simulink model "MPCRLpredict"  (R2023a)
settings: Solver=ode1  StartTime=0.0  StopTime=inf  FixedStep=0.005  RelTol=1e-3  EnableMultiTasking=on
values from neighbouring files (symbols this model uses):
  B = -100    [RLmpcTrainPredict.m]
  bp = 5e-5*2    (= 0.0001)    [Copy_of_qube2_rotpen_param.m]    (also in MPCmodelinitial.m = 5e-05)
  br = 1e-3*2    (= 0.002)    [Copy_of_qube2_rotpen_param.m]    (also in MPCmodelinitial.m = 0.001)
  g = 9.81    [Copy_of_qube2_rotpen_param.m]    (also in MPCmodelinitial.m)
  Jp = mp*Lp^2/3    (= 0.0001464408)    [Copy_of_qube2_rotpen_param.m]    (also in MPCmodelinitial.m = 0.000133128)
  Jr = mr*r^2/3    (= 0.000251670833333)    [Copy_of_qube2_rotpen_param.m]    (also in MPCmodelinitial.m = 0.000228791666667)
  km = kt    (= 0.042)    [Copy_of_qube2_rotpen_param.m]    (also in MPCmodelinitial.m)
  kt = 0.042    [Copy_of_qube2_rotpen_param.m]    (also in MPCmodelinitial.m)
  l = Lp/2    (= 0.0645)    [Copy_of_qube2_rotpen_param.m]    (also in MPCmodelinitial.m)
  mp = 0.024*1.1    (= 0.0264)    [Copy_of_qube2_rotpen_param.m]    (also in MPCmodelinitial.m = 0.024)
  q11 = 5    [RLmpcTrainPredict.m]
  q22 = 5    [RLmpcTrainPredict.m]
  q33 = 0    [RLmpcTrainPredict.m]
  q44 = 0    [RLmpcTrainPredict.m]
  r = 0.085    [Copy_of_qube2_rotpen_param.m]    (also in MPCmodelinitial.m)
  Rm = 9.7    [Copy_of_qube2_rotpen_param.m]    (also in MPCmodelinitial.m = 8.4)
  theta_max = 2    [RLmpcTrainPredict.m]
  UR = 0.1    [RLmpcTrainPredict.m]
  UVR = 0    [RLmpcTrainPredict.m]
undefined symbols (not defined in the file or in its folder): ic_alpha0
libraries: simulink x5, mpclib x1, rllib x1, sdolib x1
settings Model: ExtModeTrigDuration=10000  Creator=XIJ62  LastModifiedBy=XIJ62
settings SolverCC: AlgebraicLoopSolver=TrustRegion  PositivePriorityOrder=on
settings DataIOCC: ReturnWorkspaceOutputs=off
settings DebuggingCC: UnconnectedInputMsg=warning  UnconnectedOutputMsg=warning  UnconnectedLineMsg=warning  ArithmeticOperatorsInVariantConditions=warning
settings ModelReferenceCC: EnableRefExpFcnMdlSchedulingChecks=on
settings SFSimCC: SimUseLocalCustomCode=off  CustomCodeUndefinedFunction=UseInterfaceOnly
settings RTWCC: Description=QUARC Win64 Target Using Toolchain  SystemTargetFile=quarc_win64.tlc  TemplateMakefile=quarc_default_tmf  RTWUseLocalCustomCode=off  Toolchain=QUARC win64 | nmake (64-bit Windows)  BuildConfiguration=Faster Runs  DLArmComputeVersion=19.05
settings CodeAppCC: StateflowObjectComments=on
settings STFCustomTargetCC: SystemTargetFile=quarc_win64.tlc
settings GRTTargetCC: ParMdlRefBuildCompliant=off  CompOptLevelCompliant=off  CombineOutputUpdateFcns=off  MatFileLogging=off  CPPClassGenCompliant=off  GRTInterface=on  ExtMode=on  ExtModeMexFile=quarc_comm
settings ConfigComp: CovMetricSettings=dswe

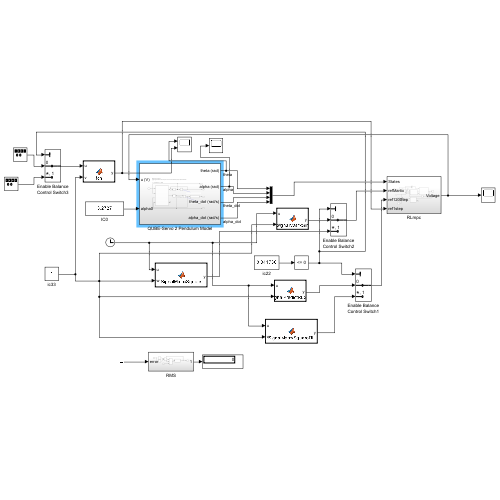
[thumbnail: Simulink's stored preview of the top-level diagram]
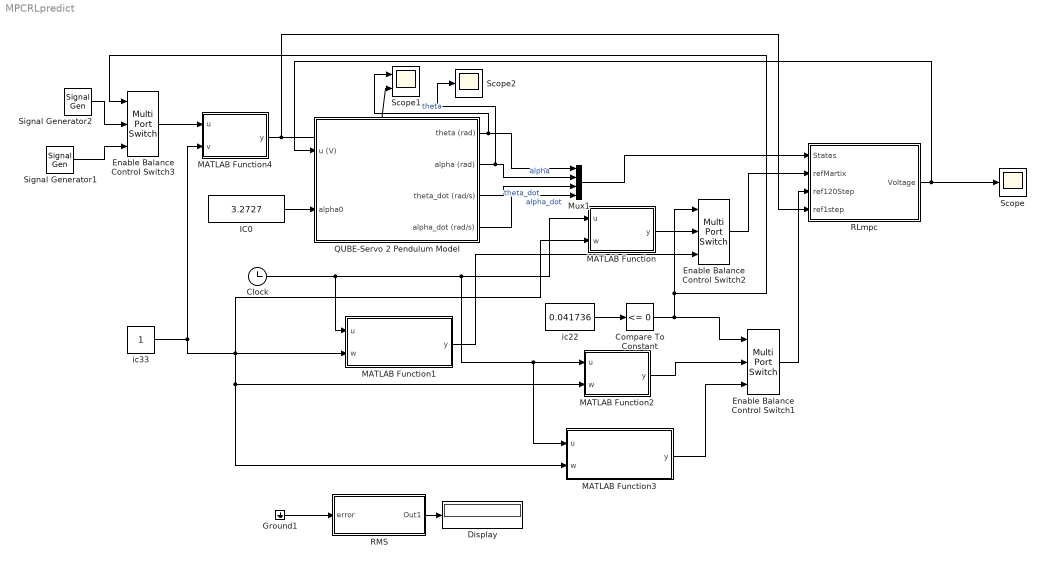
== system MPCRLpredict ==
  Clock : Clock
  Compare To Constant : simulink/Logic and Bit Operations/Compare To Constant  relop=<=  const=0  OutDataTypeStr=boolean
  Display : Display
  Enable Balance Control Switch1 : MultiPortSwitch  DataPortOrder=Zero-based contiguous  Inputs=2  zeroidx=on  SaturateOnIntegerOverflow=off  InputSameDT=off
  Enable Balance Control Switch2 : MultiPortSwitch  DataPortOrder=Zero-based contiguous  Inputs=2  zeroidx=on  SaturateOnIntegerOverflow=off  InputSameDT=off
  Enable Balance Control Switch3 : MultiPortSwitch  DataPortOrder=Zero-based contiguous  Inputs=2  zeroidx=on  SaturateOnIntegerOverflow=off  InputSameDT=off
  Ground1 : Ground
  IC0 : Constant  Value=3.2727
  MATLAB Function : MATLAB Function  TreatAsAtomicUnit=on
  MATLAB Function1 : MATLAB Function  TreatAsAtomicUnit=on
  MATLAB Function2 : MATLAB Function  TreatAsAtomicUnit=on
  MATLAB Function3 : MATLAB Function  TreatAsAtomicUnit=on
  MATLAB Function4 : MATLAB Function  TreatAsAtomicUnit=on
  Mux1 : Mux
  QUBE-Servo 2 Pendulum Model : Subsystem
  RLmpc : Subsystem
  RMS : Subsystem
  Scope : Scope
  Scope1 : Scope  NumInputPorts=2
  Scope2 : Scope
  Signal Generator1 : SignalGenerator  WaveForm=square  Amplitude=0.5  Units=rad/sec
  Signal Generator2 : SignalGenerator  Units=rad/sec
  ic22 : Constant  Value=0.041736
  ic33 : Constant
  wires:
  RLmpc/1(Voltage) -> Scope/1, QUBE-Servo 2 Pendulum Model/1(u (V))
  Signal Generator1/1 -> Enable Balance Control Switch3/3
  Clock/1 -> MATLAB Function/1(u), MATLAB Function3/1(u), MATLAB Function2/1(u), MATLAB Function1/1(u)
  MATLAB Function1/1(y) -> Enable Balance Control Switch2/3
  QUBE-Servo 2 Pendulum Model/1(theta (rad)) -> Scope1/1, Mux1/1  "theta"
  QUBE-Servo 2 Pendulum Model/2(alpha (rad)) -> Scope2/1, Mux1/2  "alpha"
  QUBE-Servo 2 Pendulum Model/3(theta_dot (rad/s)) -> Mux1/3  "theta_dot"
  QUBE-Servo 2 Pendulum Model/4(alpha_dot (rad/s)) -> Mux1/4  "alpha_dot"
  Mux1/1 -> RLmpc/1(States)
  IC0/1 -> QUBE-Servo 2 Pendulum Model/2(alpha0)
  RMS/1(Out1) -> Display/1
  Ground1/1 -> RMS/1(error)
  MATLAB Function2/1(y) -> Enable Balance Control Switch1/2
  Enable Balance Control Switch1/1 -> RLmpc/3(ref120Step)
  MATLAB Function3/1(y) -> Enable Balance Control Switch1/3
  Compare To Constant/1 -> Enable Balance Control Switch3/1, Enable Balance Control Switch2/1, Enable Balance Control Switch1/1
  ic22/1 -> Compare To Constant/1
  MATLAB Function/1(y) -> Enable Balance Control Switch2/2
  Enable Balance Control Switch2/1 -> RLmpc/2(refMartix)
  Signal Generator2/1 -> Enable Balance Control Switch3/2
  ic33/1 -> MATLAB Function4/2(v), MATLAB Function3/2(w), MATLAB Function2/2(w), MATLAB Function1/2(w), MATLAB Function/2(w)
  Enable Balance Control Switch3/1 -> MATLAB Function4/1(u)
  MATLAB Function4/1(y) -> Scope1/2, RLmpc/4(ref1step)

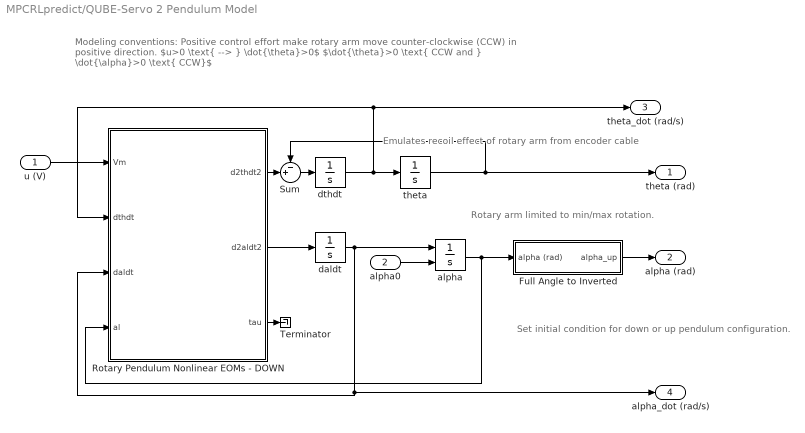
== system MPCRLpredict/QUBE-Servo 2 Pendulum Model ==
  note: Rotary arm limited to min/max rotation.
  note: Modeling conventions:
      | Positive control effort make rotary arm move counter-clockwise (CCW) in positive direction.
      | $u>0 \text{ --> } \dot{\theta}>0$
      | $\dot{\theta}>0 \text{ CCW and } \dot{\alpha}>0 \text{ CCW}$
  note: Set initial condition for down or up pendulum configuration.
  note: Emulates recoil effect of rotary arm from encoder cable
  u (V) : Inport
  alpha0 : Inport  Port=2
  Full Angle to Inverted : Subsystem
  Rotary Pendulum Nonlinear EOMs - DOWN : MATLAB Function  TreatAsAtomicUnit=on
  Sum : Sum  Inputs=-+|
  Terminator : Terminator
  alpha : Integrator  InitialConditionSource=external  InitialCondition=ic_alpha0
  daldt : Integrator
  dthdt : Integrator
  theta : Integrator  LimitOutput=on  UpperSaturationLimit=theta_max  LowerSaturationLimit=-theta_max
  theta (rad) : Outport  VectorParamsAs1DForOutWhenUnconnected=off
  alpha (rad) : Outport  Port=2  VectorParamsAs1DForOutWhenUnconnected=off
  theta_dot (rad/s) : Outport  Port=3  VectorParamsAs1DForOutWhenUnconnected=off
  alpha_dot (rad/s) : Outport  Port=4  VectorParamsAs1DForOutWhenUnconnected=off
  wires:
  daldt/1 -> Rotary Pendulum Nonlinear EOMs - DOWN/3(daldt), alpha_dot (rad/s)/1, alpha/1
  alpha/1 -> Full Angle to Inverted/1(alpha (rad)), Rotary Pendulum Nonlinear EOMs - DOWN/4(al)
  Rotary Pendulum Nonlinear EOMs - DOWN/2(d2aldt2) -> daldt/1
  dthdt/1 -> theta_dot (rad/s)/1, Rotary Pendulum Nonlinear EOMs - DOWN/2(dthdt), theta/1
  u (V)/1 -> Rotary Pendulum Nonlinear EOMs - DOWN/1(Vm)
  Rotary Pendulum Nonlinear EOMs - DOWN/3(tau) -> Terminator/1
  Full Angle to Inverted/1(alpha_up) -> alpha (rad)/1
  alpha0/1 -> alpha/2
  theta/1 -> theta (rad)/1, Sum/1
  Rotary Pendulum Nonlinear EOMs - DOWN/1(d2thdt2) -> Sum/2
  Sum/1 -> dthdt/1

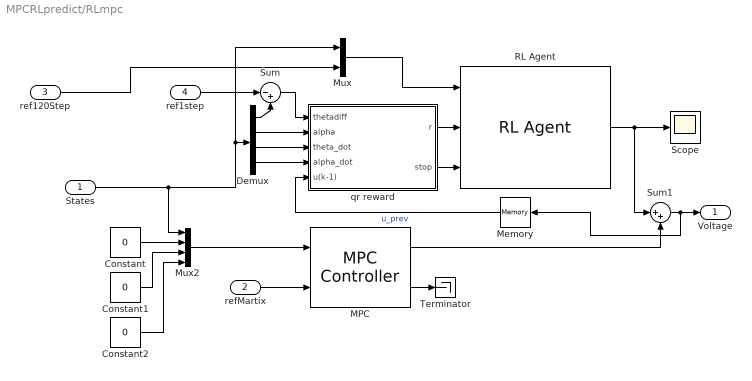
== system MPCRLpredict/RLmpc ==
  States : Inport
  refMartix : Inport  Port=2
  ref120Step : Inport  Port=3
  ref1step : Inport  Port=4
  Constant : Constant  Value=0
  Constant1 : Constant  Value=0
  Constant2 : Constant  Value=0
  Demux : Demux
  MPC : mpclib/MPC Controller  SCDEnableBlockLinearizationSpecification=on  mpcobj=mpc1  is_multiple=0  enable_value=0  return_u0=off  updateMPCinCallerWorkspace=on  md_inport=off  mv_inport=off  uref_inport=off  return_cost=off  return_mvseq=off  return_qpstatus=off  return_xseq=off  return_state=on  return_ovseq=off  state_inport=on  umin_inport=off  umax_inport=off  ymin_inport=off  ymax_inport=off  cc_inport=off  ywt_inport=off  uwt_inport=off  duwt_inport=off  rhoeps_inport=off  pm_inport=off  MaximumP=10  HorizonChoice=FixedHorizon  n_ts=0.005  n_p=120  n_mv=1  n_md=0  n_ud=0  n_mo=4  n_uo=0  BlockDataType=double  SampleTimeInherited=off  switch_inport=off
  Memory : Memory
  Mux : Mux  Inputs=2
  Mux2 : Mux
  RL Agent : rllib/RL Agent  Agent=agent  ExternalActionAsInput=off  ProvideLastAction=off  ProvideCumRwd=off  TreatAsDirectFeedthrough=on  UseStrictObservationDataTypes=off
  Scope : Scope
  Sum : Sum  Inputs=|-+
  Sum1 : Sum  Inputs=|++
  Terminator : Terminator
  qr reward : Subsystem
  Voltage : Outport
  wires:
  States/1 -> Mux2/1, Mux/1, Demux/1
  refMartix/1 -> MPC/2
  qr reward/2(stop) -> RL Agent/3
  qr reward/1(r) -> RL Agent/2
  Demux/2 -> qr reward/2(alpha)
  Demux/3 -> qr reward/3(theta_dot)
  Demux/4 -> qr reward/4(alpha_dot)
  Demux/1 -> Sum/2
  Sum/1 -> qr reward/1(thetadiff)
  Mux/1 -> RL Agent/1
  RL Agent/1 -> Sum1/1, Scope/1
  Memory/1 -> qr reward/5(u(k-1))  "u_prev"
  MPC/2 -> Terminator/1
  MPC/1 -> Sum1/2
  Sum1/1 -> Memory/1, Voltage/1
  Constant1/1 -> Mux2/3
  Constant2/1 -> Mux2/4
  Constant/1 -> Mux2/2
  Mux2/1 -> MPC/1
  ref120Step/1 -> Mux/2
  ref1step/1 -> Sum/1

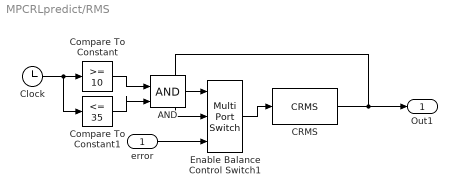
== system MPCRLpredict/RMS ==
  error : Inport
  AND : Logic  IconShape=distinctive  AllPortsSameDT=off  OutDataTypeStr=boolean
  CRMS : sdolib/RMS Blocks/CRMS
  Clock : Clock
  Compare To Constant : simulink/Logic and Bit Operations/Compare To Constant  relop=>=  const=10  OutDataTypeStr=boolean
  Compare To Constant1 : simulink/Logic and Bit Operations/Compare To Constant  relop=<=  const=35  OutDataTypeStr=boolean
  Enable Balance Control Switch1 : MultiPortSwitch  DataPortOrder=Zero-based contiguous  Inputs=2  zeroidx=on  SaturateOnIntegerOverflow=off  InputSameDT=off
  Out1 : Outport
  wires:
  Clock/1 -> Compare To Constant/1, Compare To Constant1/1
  Compare To Constant1/1 -> AND/2
  Compare To Constant/1 -> AND/1
  AND/1 -> Enable Balance Control Switch1/1
  Enable Balance Control Switch1/1 -> CRMS/1
  CRMS/1 -> Enable Balance Control Switch1/2, Out1/1
  error/1 -> Enable Balance Control Switch1/3

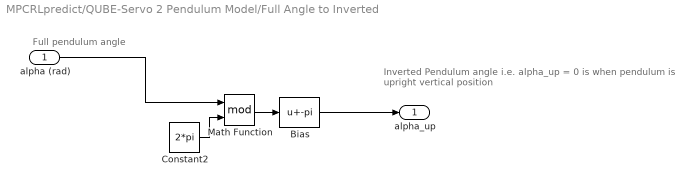
== system MPCRLpredict/QUBE-Servo 2 Pendulum Model/Full Angle to Inverted ==
  note: Inverted Pendulum angle
      | i.e. alpha_up = 0 is when pendulum is upright vertical position
  note: Full pendulum angle
  alpha (rad) : Inport
  Bias : Bias  Bias=-pi  SaturateOnIntegerOverflow=off
  Constant2 : Constant  Value=2*pi
  Math Function : Math  Operator=mod  SignedPower=on
  alpha_up : Outport  VectorParamsAs1DForOutWhenUnconnected=off
  wires:
  Constant2/1 -> Math Function/2
  Bias/1 -> alpha_up/1
  alpha (rad)/1 -> Math Function/1
  Math Function/1 -> Bias/1

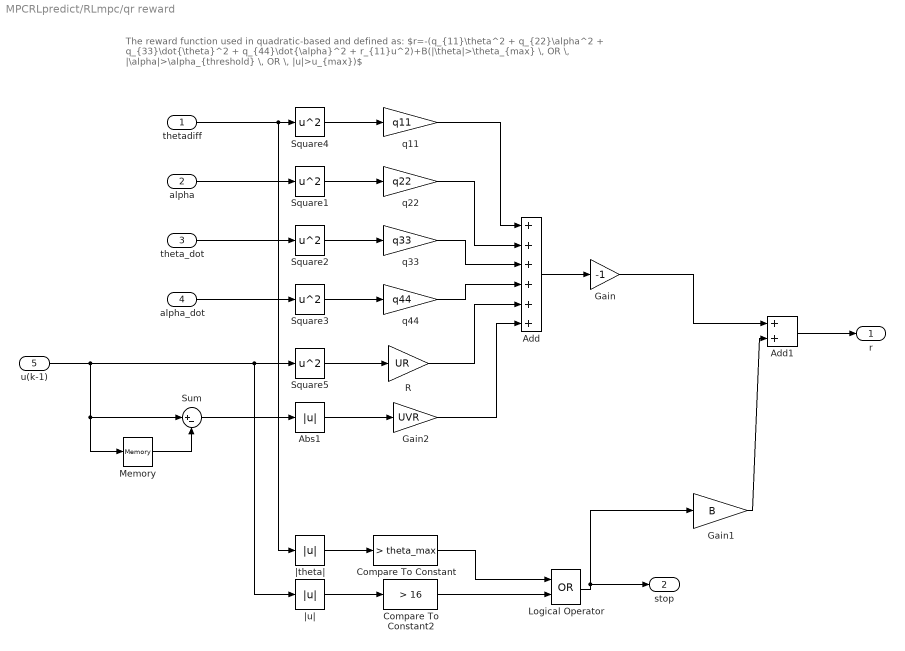
== system MPCRLpredict/RLmpc/qr reward ==
  note: The reward function used in quadratic-based and defined as:
      | $r=-(q_{11}\theta^2 + q_{22}\alpha^2 + q_{33}\dot{\theta}^2 + q_{44}\dot{\alpha}^2 + r_{11}u^2)+B(|\theta|>\theta_{max} \, OR \, |\alpha|>\alpha_{threshold} \, OR \, |u|>u_{max})$
  thetadiff : Inport
  alpha : Inport  Port=2
  theta_dot : Inport  Port=3
  alpha_dot : Inport  Port=4
  u(k-1) : Inport  Port=5
  Abs1 : Abs  SaturateOnIntegerOverflow=off
  Add : Sum  Inputs=++++++
  Add1 : Sum
  Compare To Constant : simulink/Logic and Bit Operations/Compare To Constant  relop=>  const=theta_max  OutDataTypeStr=boolean
  Compare To Constant2 : simulink/Logic and Bit Operations/Compare To Constant  relop=>  const=16  OutDataTypeStr=boolean
  Gain : Gain  Gain=-1
  Gain1 : Gain  Gain=B
  Gain2 : Gain  Gain=UVR
  Logical Operator : Logic  Operator=OR  AllPortsSameDT=off  OutDataTypeStr=boolean
  Memory : Memory
  R : Gain  Gain=UR
  Square{1..5} (5 alike) : Math  Operator=square
  Sum : Sum  Inputs=|+-
  q11 : Gain  Gain=q11
  q22 : Gain  Gain=q22
  q33 : Gain  Gain=q33
  q44 : Gain  Gain=q44
  |theta| : Abs  SaturateOnIntegerOverflow=off
  |u| : Abs  SaturateOnIntegerOverflow=off
  r : Outport  VectorParamsAs1DForOutWhenUnconnected=off
  stop : Outport  Port=2  VectorParamsAs1DForOutWhenUnconnected=off
  wires:
  |theta|/1 -> Compare To Constant/1
  thetadiff/1 -> Square4/1, |theta|/1
  Compare To Constant/1 -> Logical Operator/1
  alpha/1 -> Square1/1
  Logical Operator/1 -> Gain1/1, stop/1
  Square4/1 -> q11/1
  Square1/1 -> q22/1
  Square2/1 -> q33/1
  theta_dot/1 -> Square2/1
  alpha_dot/1 -> Square3/1
  Square3/1 -> q44/1
  u(k-1)/1 -> Square5/1, |u|/1, Sum/1, Memory/1
  Square5/1 -> R/1
  |u|/1 -> Compare To Constant2/1
  R/1 -> Add/5
  q11/1 -> Add/1
  q33/1 -> Add/3
  q22/1 -> Add/2
  q44/1 -> Add/4
  Add/1 -> Gain/1
  Compare To Constant2/1 -> Logical Operator/2
  Gain/1 -> Add1/1
  Gain1/1 -> Add1/2
  Add1/1 -> r/1
  Memory/1 -> Sum/2
  Sum/1 -> Abs1/1
  Abs1/1 -> Gain2/1
  Gain2/1 -> Add/6

== matlab function MPCRLpredict/MATLAB Function1 ==
  data: u input; y output; w input
function y = SignalMatrixSquare(u,w)
    Signal=zeros(120,4);
    for (k=1:120)
        t=floor((u+0.005*k-0.005)/pi);
        Signal(k,1)=mod(t,2)-0.5;
    end
    y = Signal*w;
end

== matlab function MPCRLpredict/MATLAB Function ==
  data: u input; y output; w input
function y = SignalMatrixSin(u,w)
    Np=120; %Prediction horizon
    Signal=zeros(120,4);
    t=u;
    for (k=1:120)
        Signal(k,1)=sin(t+0.005*k-0.005);
    end
    y = Signal*w;
end

== matlab function MPCRLpredict/MATLAB Function2 ==
  data: u input; y output; w input
function y = SignalPredictRLSin(u,w)
    Np=120; %Prediction horizon
    Signal=zeros(120,1);
    t=u;
    for (k=1:120)
        Signal(k)=sin(t+0.005*k-0.005);
    end
    y = Signal*w;
end

== matlab function MPCRLpredict/MATLAB Function3 ==
  data: u input; y output; w input
function y = SignalMatrixSquareRL(u,w)
    Signal=zeros(120,1);
    for (k=1:120)
        t=floor((u+0.005*k-0.005)/pi);
        Signal(k)=mod(t,2)-0.5;
    end
    y = Signal*w;
end

== matlab function MPCRLpredict/MATLAB Function4 ==
  data: u input; y output; v input
function y = fcn(u,v)
    
    
y=u*v;

== matlab function MPCRLpredict/QUBE-Servo 2 Pendulum Model/Rotary Pendulum Nonlinear EOMs - DOWN ==
  data: Vm input size=1; d2thdt2 output size=1; d2aldt2 output size=1; dthdt input size=1; daldt input size=1; Jp parameter; Jr parameter; l parameter; mp parameter; br parameter; bp parameter; r parameter; kt parameter; km parameter; Rm parameter; al input size=1; g parameter; tau output
function [d2thdt2,d2aldt2,tau] = pen_nonlin_eoms(Vm, dthdt, daldt, Jp, Jr, l, mp, br, bp, r, kt, km, Rm, al, g)

% Convert voltage to torque input
tau = (Vm - km*dthdt)/Rm;
tau=kt*tau;
% Denominator
Jt = Jr*Jp + Jp^2*sin(al)^2 - mp^2*r^2*l^2*cos(al)^2;
% Nonlinear equations of motion for generic rotary pendulum (i.e. furuta)
% Terms from EOM solving
term1 = tau - br*dthdt + 2*Jp*sin(al)*cos(al)*dthdt*daldt + mp*r*l*sin(al)*daldt^2;
term2 = -bp*daldt - Jp*sin(al)*cos(al)*daldt^2 - mp*g*l*sin(al);
% Torque to rotary arm position)
d2thdt2 = 1/Jt*( Jp*term1 - mp*r*l*cos(al)*term2);
% Torque to pendulum angle position
d2aldt2 = 1/Jt*(-mp*r*l*cos(al)*term1 + (Jr+Jp*sin(al)^2)*term2);
